simulink model "Host_serial_final"  (Simulink 8.2)
settings: Solver=ode23t  StartTime=0.0  StopTime=10  RelTol=1e-3
InitFcn:
  | tstop = str2num(get_param(bdroot,'StopTime'));
StopFcn:
  | instrreset
undefined symbols (not defined in the file or in its folder): NULL, serial, sigbuilder_block
libraries: instrumentlib x3, demoLibrary x1, aerolibanimutils x1
settings Model: Creator=deastman  LastModifiedBy=pvinnako
settings DataIOCC: LimitDataPoints=off  SignalLoggingSaveFormat=Dataset  SaveOutput=off  SaveTime=off
settings DebuggingCC: SolverPrmCheckMsg=none  ParameterOverflowMsg=warning  FcnCallInpInsideContextMsg=EnableAllAsWarning  StrictBusMsg=Warning
settings ConfigurationSet: Description=SimMechanics 2G

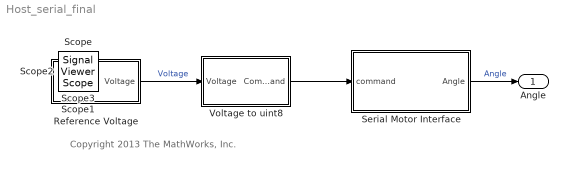
== system Host_serial_final ==
  note: Copyright 2013 The MathWorks, Inc.
  Reference Voltage : Subsystem  Tag=STV Subsys  LoadFcn=sigbuilder_block('load');  StartFcn=sigbuilder_block('start');  StopFcn=sigbuilder_block('stop');  ClipboardFcn=sigbuilder_block('clipboard');  mask(Sigbuilder block){}
      mask help: Sigbuilder GUI
      mask init:
      | if ~strcmp(get_param(bdroot(gcbh),'SimulationStatus'),'stopped') tuvar = sigbuilder_block('maskInit'); end
      settings: CopyFcn=sigbuilder_block('copy');  DeleteFcn=sigbuilder_block('delete');  ModelCloseFcn=sigbuilder_block('modelClose');  PreSaveFcn=sigbuilder_block('preSave');  PauseFcn=sigbuilder_block('pause')  ContinueFcn=sigbuilder_block('continue')  NameChangeFcn=sigbuilder_block('namechange');  OpenFcn=sigbuilder_block('open',[135 60.75 1183.5 252 ]);  CloseFcn=sigbuilder_block('close');
      mask Display: plot(0,0,100,100,[10,10,40,40,10],[80,20,20,80,80],[40,10],[50,50], [40,27,10],[65,72,56],[40,25,25,10],[28,28,43,43]);
  Serial Motor Interface : Subsystem
  Voltage to uint8 : Subsystem
  Angle : Outport
  Scope : SignalViewerScope  IOType=viewer  NumInputPorts=2  RefreshTime=0.035000
      settings: TimeRange=10  YMin=-3~-150  YMax=3~100
  Scope1 : SignalViewerScope  IOType=viewer  NumInputPorts=2  ZoomMode=xonly  LegendLocations="0.73608     0.95519     0.22542    0.033553   0.753      0.4944     0.20384    0.033553"  RefreshTime=0.035000
      settings: ShowLegends=on  TimeRange=10  YMin=-1~-120  YMax=1~80  SaveName=ScopeData3
  Scope2 : SignalViewerScope  IOType=viewer  RefreshTime=0.035000
  Scope3 : SignalViewerScope  IOType=viewer  RefreshTime=0.035000
      settings: SaveName=ScopeData2
  wires:
  Reference Voltage/1(Voltage) -> Voltage to uint8/1(Voltage)  "Voltage"
  Serial Motor Interface/1(Angle) -> Angle/1  "Angle"
  Voltage to uint8/1(Command) -> Serial Motor Interface/1(command)

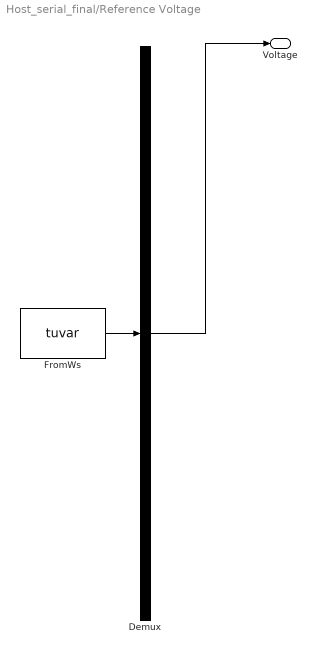
== system Host_serial_final/Reference Voltage ==
  Demux : Demux  Tag=STV Demux  Outputs=1
  FromWs : FromWorkspace  Tag=STV FromWs  VariableName=tuvar  SampleTime=1/100  SigBuilderData=DataTag0  VnvData=DataTag1
      SigBuilderData=|
      | common.afterFinalStr = 'Extrapolate'
      | common.sampleTime = '1/100'
      | dataSet(1).timeRange = [0 10]
      | dataSet(1).name = 'Bounds1_z11'
      | dataSet(2).timeRange = [0 10]
      | dataSet(2).name = 'Bounds5_z4'
      | dataSet(3).timeRange = [0 20]
      | dataSet(3).name = 'Sine3_z1'
      | dataSet(4).timeRange = [0 20]
      | dataSet(4).name = 'Sine5_z2'
      | dataSet(5).timeRange = [0 20]
      | dataSet(5).name = 'Step1_z5'
      | dataSet(6).timeRange = [0 20]
      | dataSet(6).name = 'Step2_z8'
      | dataSet(7).timeRange = [0 10]
      | dataSet(7).name = 'RampSquare_z3'
      | dataSet(8).timeRange = [0 10]
      | dataSet(8).name = 'Steps_z9'
      | dataSet(9).timeRange = [0 10]
      | dataSet(9).name = 'Small Steps_z6'
      | dataSet(10).timeRange = [0 10]
      | dataSet(10).name = 'Square_z10'
      | dataSet(11).timeRange = [0 55]
      | dataSet(11).name = 'DeadZone_z7'
      | sbobj.Groups(1).Name = 'Bounds1_z11'
      | sbobj.Groups(1).Signals.Name = 'Voltage'
      | sbobj.Groups(1).Signals.XData = [0 2.5 2.5 5 5 7.5 7.5 10]
      | sbobj.Groups(1).Signals.YData = [1 1 -1 -1 1 1 -1 -1]
      | sbobj.Groups(2).Name = 'Bounds5_z4'
      | sbobj.Groups(2).Signals.Name = 'Voltage'
      | sbobj.Groups(2).Signals.XData = [0 2.5 2.5 5 5 7.5 7.5 10]
      | sbobj.Groups(2).Signals.YData = [5 5 -5 -5 5 5 -5 -5]
      | sbobj.Groups(3).Name = 'Sine3_z1'
      | sbobj.Groups(3).Signals.Name = 'Voltage'
      | sbobj.Groups(3).Signals.XData = [0 0.01 0.02 0.03 0.04 0.05 0.06 0.07 0.08 0.09 0.1 0.11 ... (2001 elements, 1x2001)]
      | sbobj.Groups(3).Signals.YData = [0 0.0299995000025 0.05999600008 0.0899865006075 0.11996800256 0.149937507812 0.179892019438 0.209828542013 0.239744081908 0.269635647594 0.29950024994 0.329334902512 ... (2001 elements, 1x2001)]
      | sbobj.Groups(3).TimeRange = [0 20]
      | sbobj.Groups(4).Name = 'Sine5_z2'
      | sbobj.Groups(4).Signals.Name = 'Voltage'
      | sbobj.Groups(4).Signals.XData = [0 0.01 0.02 0.03 0.04 0.05 0.06 0.07 0.08 0.09 0.1 0.11 ... (2001 elements, 1x2001)]
      | sbobj.Groups(4).Signals.YData = [0 0.0499991666708 0.0999933334667 0.149977501012 0.199946670933 0.249895846353 0.299820032397 0.349714236688 0.399573469846 0.44939274599 0.499167083234 0.548891504186 ... (2001 elements, 1x2001)]
      | sbobj.Groups(4).TimeRange = [0 20]
      | sbobj.Groups(5).Name = 'Step1_z5'
      | sbobj.Groups(5).Signals.Name = 'Voltage'
      | sbobj.Groups(5).Signals.XData = [0 0.01 0.02 0.03 0.04 0.05 0.06 0.07 0.08 0.09 0.1 0.11 ... (2001 elements, 1x2001)]
      | sbobj.Groups(5).Signals.YData = [0 0 0 0 0 0 0 0 0 0 0 0 ... (2001 elements, 1x2001)]
      | sbobj.Groups(5).TimeRange = [0 20]
      | sbobj.Groups(6).Name = 'Step2_z8'
      | sbobj.Groups(6).Signals.Name = 'Voltage'
      | sbobj.Groups(6).Signals.XData = [0 0.01 0.02 0.03 0.04 0.05 0.06 0.07 0.08 0.09 0.1 0.11 ... (2001 elements, 1x2001)]
      | sbobj.Groups(6).Signals.YData = [0 0 0 0 0 0 0 0 0 0 0 0 ... (2001 elements, 1x2001)]
      | sbobj.Groups(6).TimeRange = [0 20]
      | sbobj.Groups(7).Name = 'RampSquare_z3'
      | sbobj.Groups(7).Signals.Name = 'Voltage'
      | sbobj.Groups(7).Signals.XData = [0 1 1 2 2 3 3 4 4 5 5 6 6 7 7 8 8 9 9 9.8 9.8 10]
      | sbobj.Groups(7).Signals.YData = [0 0.75 0 -0.75 0 1.5 0 -1.5 2 2 -2 -2 3 3 -3 -3 1 1 -1 -1 0 0]
      | sbobj.Groups(8).Name = 'Steps_z9'
      | sbobj.Groups(8).Signals.Name = 'Voltage'
      | sbobj.Groups(8).Signals.XData = [0 1.52 1.52 2.4 2.4 3.66 3.68 4.64 4.64 6.02 6.02 7 7 8.96 8.96 10]
      | sbobj.Groups(8).Signals.YData = [2 2 -3 -3 3 -1 1.95 1.95 -2 -2 0.7 0.7 -1.05 -0.05 0 0]
      | sbobj.Groups(9).Name = 'Small Steps_z6'
      | sbobj.Groups(9).Signals.Name = 'Voltage'
      | sbobj.Groups(9).Signals.XData = [0 0.5 0.5 1.02 1.02 2 2 2.58 2.58 3.78 3.78 4.64 4.64 5.28 5.28 6 6 7 7 9 9 10]
      | sbobj.Groups(9).Signals.YData = [0.4 0.4 0.75 0.75 1.5 3 1.55 1.55 3.55 3.55 -3.05 -3.05 -1 -1 -0.45 -0.45 0.7 0.7 -2.05 -0.05 1 1]
      | sbobj.Groups(10).Name = 'Square_z10'
      | sbobj.Groups(10).Signals.Name = 'Voltage'
      | sbobj.Groups(10).Signals.XData = [0 0.5 0.5 1.02 1.02 1.5 1.5 2 2 2.5 2.5 3 3 4 4 5 5 6 6 7 7 8 8 9 9 9.8 9.8 10]
      | sbobj.Groups(10).Signals.YData = [0.4 0.4 -0.4 -0.4 1 1 -1 -1 1.5 1.5 -1.5 -1.5 2 2 -2 -2 3 3 -3 -3 1.3 1.3 -1.3 -1.3 -4 -4 0 0]
      | sbobj.Groups(11).Name = 'DeadZone_z7'
      | sbobj.Groups(11).Signals.Name = 'Voltage'
      | sbobj.Groups(11).Signals.XData = [0 5 5 10 10 15 15 20 25 30 30 35 40 45 50 50 55]
      | sbobj.Groups(11).Signals.YData = [0 0 0.16 0.16 0.3 0.3 0.7 0.7 -0.205 -0.205 -0.355 -0.35 -0.605 -0.605 0.005 0 0]
      | sbobj.Groups(11).TimeRange = [0 55]
  Voltage : Outport  Tag=STV Outport
  wires:
  Demux/1 -> Voltage/1
  FromWs/1 -> Demux/1

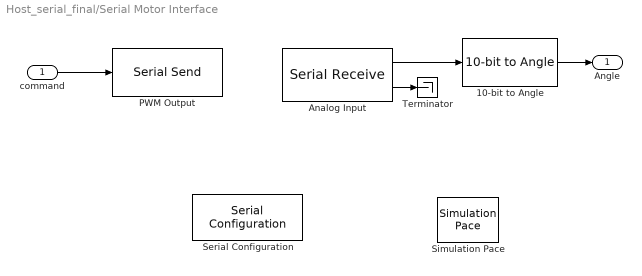
== system Host_serial_final/Serial Motor Interface ==
  command : Inport  OutDataTypeStr=uint8  SampleTime=1/10
  10-bit to Angle : demoLibrary/Utilities/10-bit to Angle
  Analog Input : instrumentlib/Serial Receive  ComPortMenu=<Please select a port...>  ComPort=COM4  ObjConstructor=serial('COM4');  Header=A  Terminator=NULL ('\0')  DataSize=1  DataType=uint16  EnableBlockingMode=off  ActionDataUnavailable=Output last received value  CustomValue=0  SampleTime=1/100
  PWM Output : instrumentlib/Serial Send  ComPortMenu=<Please select a port...>  ComPort=COM4  ObjConstructor=serial('COM4');  Terminator=<none>  EnableBlockingMode=on
  Serial Configuration : instrumentlib/Serial Configuration  Priority=-200000  ComPortMenu=<Please select a port...>  ComPort=COM4  ObjConstructor=serial('COM4');  BaudRate=9600  DataBits=8  Parity=none  StopBits=1  FlowControl=none  Timeout=1  ByteOrder=BigEndian
  Simulation Pace : aerolibanimutils/Simulation Pace  SimulationPace=1  SleepMode=MATLAB Thread  OutputPaceError=off  SampleTime=1/30
      settings: AttributesFormatString=%<SimulationPace> sec/sec
  Terminator : Terminator
  Angle : Outport
  wires:
  Analog Input/1 -> 10-bit to Angle/1
  Analog Input/2 -> Terminator/1
  command/1 -> PWM Output/1
  10-bit to Angle/1 -> Angle/1

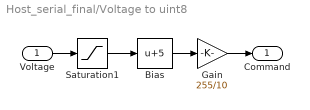
== system Host_serial_final/Voltage to uint8 ==
  Voltage : Inport
  Bias : Bias  Bias=5
  Gain : Gain  Gain=255/10  OutDataTypeStr=uint8
  Saturation1 : Saturate  UpperLimit=5  LowerLimit=-5
  Command : Outport
  wires:
  Bias/1 -> Gain/1
  Saturation1/1 -> Bias/1
  Gain/1 -> Command/1
  Voltage/1 -> Saturation1/1
